simulink model "SingleAgentMaths"  (R2017a)
settings: Solver=ode23t  StartTime=0.0  StopTime=5  FixedStep=tstep  MaxStep=tstep  RelTol=1e-3
InitFcn:
  | initSim;
StopFcn:
  | plotSimSolution;
values from neighbouring files (symbols this model uses):
  tstep = 0.01    [initSim.m]
undefined symbols (not defined in the file or in its folder): m
settings Model: Creator=yn15  LastModifiedBy=daw15
settings OptimizationCC: LifeSpan=inf
settings DebuggingCC: SFUnexpectedBacktrackingDiag=warning  SFNoUnconditionalDefaultTransitionDiag=warning  SFExecutionAtInitializationDiag=none
settings GRTTargetCC: TargetLangStandard=C89/C90 (ANSI)
settings ConfigComp: CovMetricSettings=dw  CovHtmlReporting=on  CovSaveCumulativeToWorkspaceVar=on  CovSaveSingleToWorkspaceVar=on  CovExternalEMLEnable=off

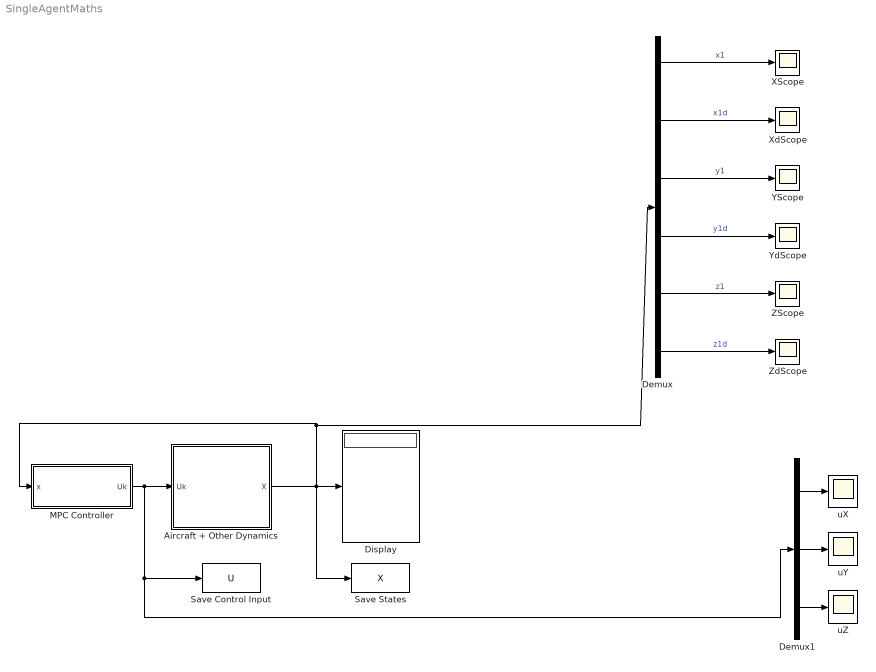
== system SingleAgentMaths ==
  Aircraft + Other Dynamics : Subsystem
  Demux : Demux  Outputs=6
  Demux1 : Demux  Outputs=3
  Display : Display
  "MPC Controller " : Subsystem
  Save Control Input : ToWorkspace  VariableName=U  SampleTime=-1
      settings: Save2DSignal=2-D array (concatenate along first dimension)
  Save States : ToWorkspace  VariableName=X  SaveFormat=Timeseries  SampleTime=-1
  XScope : Scope
  XdScope : Scope
  YScope : Scope
  YdScope : Scope
  ZScope : Scope
  ZdScope : Scope
  uX : Scope
  uY : Scope
  uZ : Scope
  wires:
  Aircraft + Other Dynamics/1(X) -> Save States/1, Demux/1, "MPC Controller "/1(x), Display/1
  Demux1/1 -> uX/1
  Demux1/2 -> uY/1
  Demux1/3 -> uZ/1
  Demux/1 -> XScope/1  "x1"
  Demux/2 -> XdScope/1  "x1d"
  Demux/3 -> YScope/1  "y1"
  Demux/4 -> YdScope/1  "y1d"
  Demux/5 -> ZScope/1  "z1"
  Demux/6 -> ZdScope/1  "z1d"
  "MPC Controller "/1(Uk) -> Aircraft + Other Dynamics/1(Uk), Demux1/1, Save Control Input/1

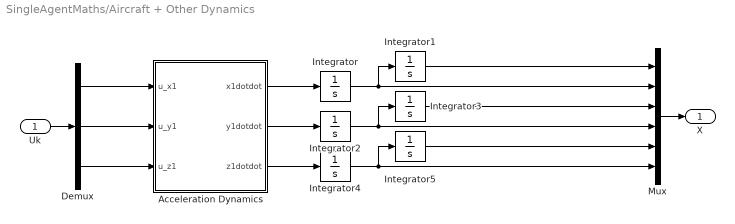
== system SingleAgentMaths/Aircraft + Other Dynamics ==
  Uk : Inport
  Acceleration Dynamics : MATLAB Function  TreatAsAtomicUnit=on
  Demux : Demux  Outputs=3
  Integrator{,2..4} (4 alike) : Integrator
  Integrator1 : Integrator  InitialCondition=2.1
  Integrator5 : Integrator  InitialCondition=2.2
  Mux : Mux  Inputs=6
  X : Outport
  wires:
  Integrator/1 -> Integrator1/1, Mux/2
  Integrator2/1 -> Mux/4, Integrator3/1
  Integrator4/1 -> Mux/6, Integrator5/1
  Integrator1/1 -> Mux/1
  Integrator3/1 -> Mux/3
  Integrator5/1 -> Mux/5
  Mux/1 -> X/1
  Uk/1 -> Demux/1
  Demux/1 -> Acceleration Dynamics/1(u_x1)
  Demux/2 -> Acceleration Dynamics/2(u_y1)
  Demux/3 -> Acceleration Dynamics/3(u_z1)
  Acceleration Dynamics/1(x1dotdot) -> Integrator/1
  Acceleration Dynamics/2(y1dotdot) -> Integrator2/1
  Acceleration Dynamics/3(z1dotdot) -> Integrator4/1

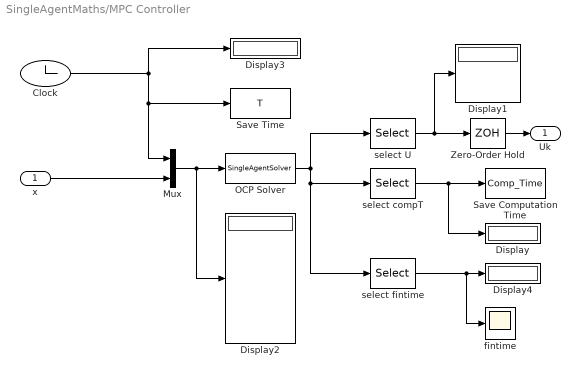
== system SingleAgentMaths/MPC Controller  ==
  x : Inport
  Clock : Clock
  Display{,1..4} (5 alike) : Display
  Mux : Mux  Inputs=2
  OCP Solver : MATLABFcn  MATLABFcn=SingleAgentSolver  OutputDimensions=m+2
  "Save Computation Time " : ToWorkspace  VariableName=Comp_Time  SampleTime=tstep
      settings: Save2DSignal=2-D array (concatenate along first dimension)
  Save Time : ToWorkspace  VariableName=T  SampleTime=-1
      settings: Save2DSignal=2-D array (concatenate along first dimension)
  Zero-Order Hold : ZeroOrderHold  SampleTime=tstep
  fintime : Scope
  select U : Selector  IndexOptions=Index vector (dialog)  Indices=3:m+2  OutputSizes=1
  select compT : Selector  IndexOptions=Index vector (dialog)  Indices=2  OutputSizes=1
  select fintime : Selector  IndexOptions=Index vector (dialog)  Indices=1  OutputSizes=1
  Uk : Outport
  wires:
  select U/1 -> Zero-Order Hold/1, Display1/1
  Clock/1 -> Save Time/1, Mux/1, Display3/1
  select compT/1 -> Display/1, "Save Computation Time "/1
  Mux/1 -> Display2/1, OCP Solver/1
  x/1 -> Mux/2
  select fintime/1 -> fintime/1, Display4/1
  OCP Solver/1 -> select U/1, select fintime/1, select compT/1
  Zero-Order Hold/1 -> Uk/1

== matlab function SingleAgentMaths/Aircraft + Other Dynamics/Acceleration Dynamics ==
  data: x1dotdot output; u_x1 input; u_y1 input; u_z1 input; y1dotdot output; z1dotdot output
function [x1dotdot,y1dotdot,z1dotdot]= dynamics(u_x1,u_y1,u_z1)

m_ag = 0.81;
gc = 9.81;

x1dotdot = (1/m_ag)*(u_x1); %x1..
y1dotdot = (1/m_ag)*(u_y1); %y1..
z1dotdot = (1/m_ag)*(u_z1 - m_ag*gc); %z1..
